simulink model "SpringMassDamper"  (R2012b)
settings: Solver=ode45  StartTime=0.0  StopTime=100.0  RelTol=1e-3
settings Model: Creator=MRDLAB  LastModifiedBy=MRDLAB

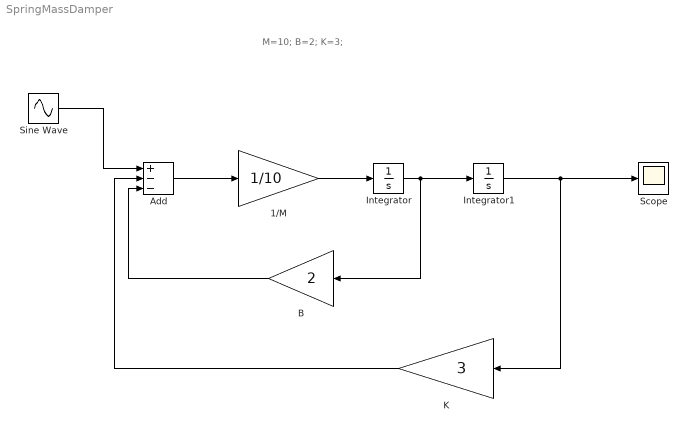
== system SpringMassDamper ==
  note: M=10;
      | B=2;
      | K=3;
  1/M : Gain  Gain=1/10
  Add : Sum  Inputs=+--
  B : Gain  Gain=2
  Integrator : Integrator
  Integrator1 : Integrator
  K : Gain  Gain=3
  Scope : Scope
  Sine Wave : Sin  SampleTime=0
  wires:
  1/M/1 -> Integrator/1
  Integrator/1 -> Integrator1/1, B/1
  Integrator1/1 -> K/1, Scope/1
  Add/1 -> 1/M/1
  B/1 -> Add/3
  K/1 -> Add/2
  Sine Wave/1 -> Add/1
